simulink model "week2prob3"  (R2020a)
settings: Solver=VariableStepAuto  StartTime=0.0  StopTime=10.0  RelTol=1e-3
PreLoadFcn:
  | b=50;
  | m=1000;
  | u=500;
  | kd=346;
  | ki=76;
  | kp=1000;
  | N=100000
settings Model: DataDictionary=week2prob3.sldd  Creator=Admin  LastModifiedBy=Admin

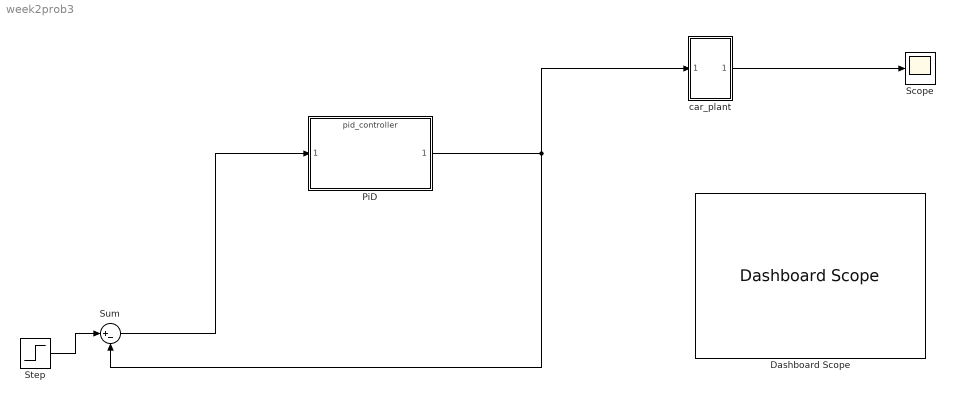
== system week2prob3 ==
  Dashboard Scope : DashboardScope
  PiD : ModelReference  ModelNameDialog=pid_controller  SimulationMode=Normal  ModelReferenceVersion=1.6
  Scope : Scope
  Step : Step  Time=0  After=u  SampleTime=0
  Sum : Sum  Inputs=|+-
  car_plant : Subsystem
  wires:
  Step/1 -> Sum/1
  PiD/1 -> car_plant/1(In1), Sum/2
  Sum/1 -> PiD/1
  car_plant/1(Out1) -> Scope/1

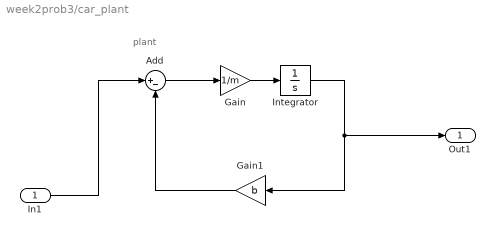
== system week2prob3/car_plant ==
  note: plant
  In1 : Inport
  Add : Sum  Inputs=|+-
  Gain : Gain  Gain=1/m
  Gain1 : Gain  Gain=b
  Integrator : Integrator
  Out1 : Outport
  wires:
  Add/1 -> Gain/1
  Gain1/1 -> Add/2
  In1/1 -> Add/1
  Gain/1 -> Integrator/1
  Integrator/1 -> Out1/1, Gain1/1
